simulink subsystem "Plant"  (R2022b)
settings: Solver=VariableStepAuto  StartTime=0.0  StopTime=10.0  RelTol=1e-3
settings Model: Creator=Mario Bertelli  LastModifiedBy=Mario Bertelli

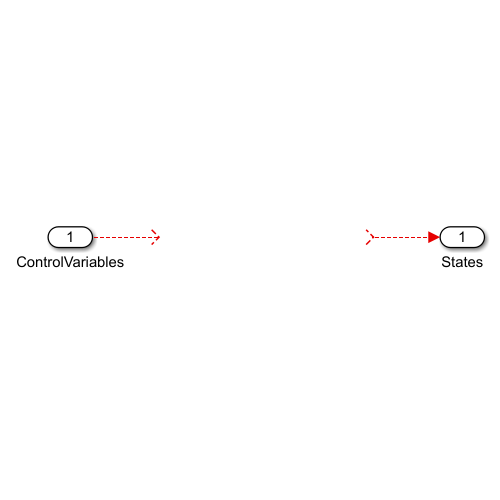
[thumbnail: Simulink's stored preview of the top-level diagram]
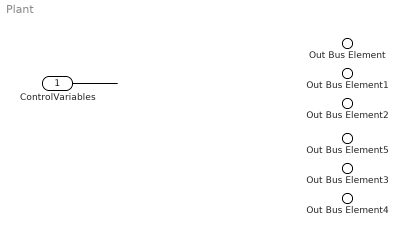
== system Plant ==
  ControlVariables : Inport
  Out Bus Element : Outport  PortName=States  Element=X
  Out Bus Element1 : Outport  PortName=States  Element=Y
  Out Bus Element2 : Outport  PortName=States  Element=Vx
  Out Bus Element3 : Outport  PortName=States  Element=Yaw
  Out Bus Element4 : Outport  PortName=States  Element=YawRate
  Out Bus Element5 : Outport  PortName=States  Element=Beta
  wires:
  ControlVariables/1 -> ?
